simulink model "tp313082"  (Simulink 3.0)
settings: Solver=ode1  StartTime=0.0  StopTime=time(end)  FixedStep=Ts/5  RelTol=1e-3
values from neighbouring files (symbols this model uses):
  Ks = input('Put identified integrator gain value Ks (0.5) = ')    [init_PI1_windupless.m]
  Ta = input('Put process time constant Ta value = (0.3) ')    [init_I0_disc2.m]    (also in step_resp1.mat = 0.3)
  Td = input('Put identified transport delay value Td (0.3) = ')    [init_PI1_windupless.m]
  u0 = 2.82328782329    [step_resp1.mat]
  u_step = 4    [step_resp1.mat]
undefined symbols (not defined in the file or in its folder): a, inp
settings Model: LastModifiedBy=mato  ExtModeTrigMode=oneshot  ExtModeArmWhenConnect=off  SaveFormat=Matrix

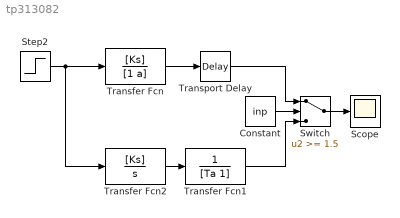
== system tp313082 ==
  Constant : Constant  Value=inp
  Scope : Scope
      settings: TimeRange=auto  YMin=-5  YMax=5  SaveName=y_sim  DataFormat=Matrix
  Step2 : Step  Time=0  Before=0  After=u_step-u0  SampleTime=0
  Switch : Switch  Threshold=1.5
  Transfer Fcn : TransferFcn  Numerator=[Ks]  Denominator=[1 a]
  Transfer Fcn1 : TransferFcn  Numerator=1  Denominator=[Ta 1]
  Transfer Fcn2 : TransferFcn  Numerator=[Ks]  Denominator=[1 0]
  Transport Delay : TransportDelay  DelayTime=Td  InitialInput=0  BufferSize=1024
  wires:
  Transfer Fcn/1 -> Transport Delay/1
  Step2/1 -> Transfer Fcn/1, Transfer Fcn2/1
  Transfer Fcn2/1 -> Transfer Fcn1/1
  Transport Delay/1 -> Switch/1
  Constant/1 -> Switch/2
  Transfer Fcn1/1 -> Switch/3
  Switch/1 -> Scope/1
